simulink model "UDPSendReceive"  (R2017b)
settings: Solver=FixedStepDiscrete  StartTime=0.0  StopTime=10.0  FixedStep=1e-3  RelTol=1e-3
libraries: mbed_lib x3, mbed_ethernet_udp x3, mbed_ethernet x1
settings Model: Creator=oh  LastModifiedBy=oh
settings OptimizationCC: DefaultParameterBehavior=Inlined
settings DebuggingCC: ParameterTunabilityLossMsg=error
settings HardwareCC: ProdBitPerPointer=32  ProdBitPerSizeT=32  ProdBitPerPtrDiffT=32  ProdLargestAtomicInteger=Long  ProdLargestAtomicFloat=Double  ProdWordSize=32  ProdHWDeviceType=ARM Compatible->ARM Cortex
settings SFSimCC: MATLABDynamicMemAlloc=off
settings RTWCC: SystemTargetFile=mbed.tlc  TemplateMakefile=mbed.tmf  Description=MbedTarget (Embedded Target for Embedded Coder)  IncludeHyperlinkInReport=on  TargetLang=C++
settings CodeAppCC: ForceParamTrailComments=on  IgnoreCustomStorageClasses=off  OperatorAnnotations=on  SimulinkDataObjDesc=on  SFDataObjDesc=on  MATLABFcnDesc=on  InsertBlockDesc=on  StateflowObjectComments=on  MATLABSourceComments=on
settings STFCustomTargetCC: TargetLibSuffix=.a  TargetLangStandard=C++03 (ISO)  GenerateSampleERTMain=on  CombineOutputUpdateFcns=on  ERTCustomFileBanners=on  SupportContinuousTime=off  SupportNonInlinedSFcns=off  RemoveResetFunc=on  MATLABClassNameForMDSCustomization=Simulink.SoftwareTarget.ERTCustomization  ModelStepFunctionPrototypeControlCompliant=on  GRTInterface=off  SystemTargetFile=mbed.tlc
settings ERTTargetCC: TargetLangStandard=C++03 (ISO)  MultiwordLength=2048  GenerateSampleERTMain=on  ParMdlRefBuildCompliant=off  CompOptLevelCompliant=off  ConcurrentExecutionCompliant=off  CPPClassGenCompliant=off  UseToolchainInfoCompliant=off  InlinedParameterPlacement=NonHierarchical  ERTCustomFileTemplate=mbed_file_process.tlc

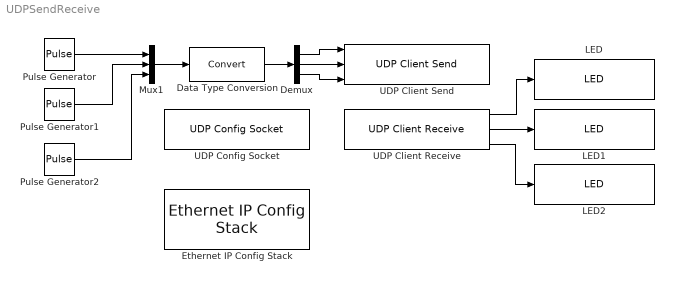
== system UDPSendReceive ==
  Data Type Conversion : DataTypeConversion
  Demux : Demux  Outputs=3
  Ethernet IP Config Stack : mbed_ethernet/Ethernet IP Config Stack  Priority=0  sDHCP=off  DHCP=0  ip_addr='192.168.178.200'  sub_mask='255.255.255.0'  gateway='0.0.0.0'
      settings: SourceProductName=Mbed Target
  LED : mbed_lib/GPIO/LED  nLED=1  SampleTime=-1
      settings: SourceProductName=Mbed Target
  LED1 : mbed_lib/GPIO/LED  nLED=2  SampleTime=-1
      settings: SourceProductName=Mbed Target
  LED2 : mbed_lib/GPIO/LED  nLED=3  SampleTime=-1
      settings: SourceProductName=Mbed Target
  Mux1 : Mux  Inputs=3
  Pulse Generator : DiscretePulseGenerator  PulseType=Time based  Period=1  PulseWidth=20
  Pulse Generator1 : DiscretePulseGenerator  PulseType=Time based  Period=1  PulseWidth=20  PhaseDelay=0.3
  Pulse Generator2 : DiscretePulseGenerator  PulseType=Time based  Period=1  PulseWidth=20  PhaseDelay=0.6
  UDP Client Receive : mbed_ethernet_udp/UDP Client Receive  sock_ID=1  caOutputPorts={'uint8' 'uint8' 'uint8'}  BufferSize=100  SampleTime=0.1
      settings: SourceProductName=Mbed Target
  UDP Client Send : mbed_ethernet_udp/UDP Client Send  sock_ID=1  caInputPorts={'uint8' 'uint8' 'uint8'}  SampleTime=0.1
      settings: SourceProductName=Mbed Target
  UDP Config Socket : mbed_ethernet_udp/UDP Config Socket  Priority=1  des_IP='192.168.178.25'  des_port=10001  sock_ID=1
      settings: SourceProductName=Mbed Target
  wires:
  UDP Client Receive/2 -> LED1/1
  UDP Client Receive/1 -> LED/1
  UDP Client Receive/3 -> LED2/1
  Pulse Generator/1 -> Mux1/1
  Pulse Generator1/1 -> Mux1/2
  Pulse Generator2/1 -> Mux1/3
  Mux1/1 -> Data Type Conversion/1
  Data Type Conversion/1 -> Demux/1
  Demux/2 -> UDP Client Send/2
  Demux/1 -> UDP Client Send/1
  Demux/3 -> UDP Client Send/3
